simulink model "EE464_HW2"  (R2021b)
settings: Solver=VariableStepAuto  StartTime=0.0  StopTime=0.001  RelTol=1e-3
libraries: spsSeriesRLCBranchLib x7, spsMosfetLib x4, spsVoltageMeasurementLib x4, spsCurrentMeasurementLib x2, spsDiodeLib x2, spsDCVoltageSourceLib x1, spsMultiWindingTransformerLib x1, spspowerguiLib x1
settings Model: Creator=Casper  LastModifiedBy=Casper

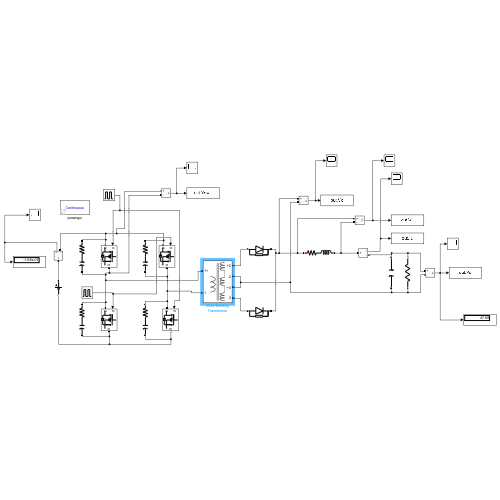
[thumbnail: Simulink's stored preview of the top-level diagram]
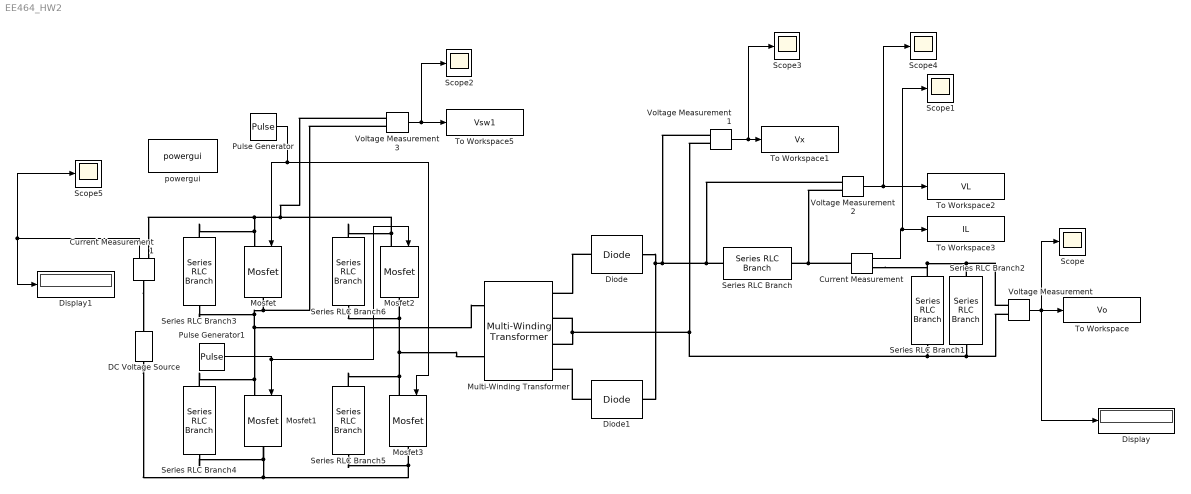
== system EE464_HW2 ==
  Current Measurement : spsCurrentMeasurementLib/Current Measurement  PhasorSimulation=off  OutputType=Complex  PSBequivalent=0
  Current Measurement1 : spsCurrentMeasurementLib/Current Measurement  PhasorSimulation=off  OutputType=Complex  PSBequivalent=0
  DC Voltage Source : spsDCVoltageSourceLib/DC Voltage Source  Amplitude=12  Measurements=None
  Diode : spsDiodeLib/Diode  Ron=0.001  Lon=0  Vf=0.001  IC=0  UseSnubber=0  Rs=500  Cs=250e-9  Measurements=off
  Diode1 : spsDiodeLib/Diode  Ron=0.001  Lon=0  Vf=0.001  IC=0  UseSnubber=0  Rs=500  Cs=250e-9  Measurements=off
  Display : Display
  Display1 : Display
  Mosfet{,1..3} (4 alike) : spsMosfetLib/Mosfet  Ron=0  Lon=0  Rd=0  Vfd=0  IC=0  Rs=inf  Cs=inf  Measurements=off
  Multi-Winding Transformer : spsMultiWindingTransformerLib/Multi-Winding Transformer  LeftWindings=1  RightWindings=2  TappedWindings=no taps  NumberOfTaps=2  SetSaturation=off  Hysteresis=off  DataFile='hysteresis.mat'  Measurements=None  UNITS=SI  NominalPower=[96 100e3]  NominalVoltages="[ 12  60  60 60 ]"  WindingResistances=[0 0 0 0]  WindingInductances=[0 0 0 0]  Rm=Inf  Lm=Inf  Saturation=[0 0;0.3072 8.754e-10;128 1.1088e-09]  BreakLoop=off  DiscreteSolver=Trapezoidal iterative  DataType=on  InitialFlux=0  TransfoNumber=1
      settings: SourceProductBaseCode=PS
  Pulse Generator : DiscretePulseGenerator  PulseType=Time based  Period=1e-5  PulseWidth=40
  Pulse Generator1 : DiscretePulseGenerator  PulseType=Time based  Period=1e-5  PulseWidth=40  PhaseDelay=5e-6
  Scope{,1..5} (6 alike) : Scope
  Series RLC Branch : spsSeriesRLCBranchLib/Series RLC Branch  LConnTagsString=__new0  RConnTagsString=__new0  BranchType=RL  Resistance=1e-10  Inductance=240e-6  SetiL0=off  InitialCurrent=0  Capacitance=1e-6  Setx0=off  InitialVoltage=0  Measurements=None
  Series RLC Branch1 : spsSeriesRLCBranchLib/Series RLC Branch  LConnTagsString=__new0  RConnTagsString=__new0  BranchType=C  Resistance=1  Inductance=1e-3  SetiL0=off  InitialCurrent=0  Capacitance=260.4e-9  Setx0=off  InitialVoltage=0  Measurements=None
  Series RLC Branch2 : spsSeriesRLCBranchLib/Series RLC Branch  LConnTagsString=__new0  RConnTagsString=__new0  BranchType=R  Resistance=24  Inductance=1e-3  SetiL0=off  InitialCurrent=0  Capacitance=1e-6  Setx0=off  InitialVoltage=0  Measurements=None
  Series RLC Branch{3..6} (4 alike) : spsSeriesRLCBranchLib/Series RLC Branch  LConnTagsString=__new0  RConnTagsString=__new0  BranchType=RC  Resistance=0.01  Inductance=1e-3  SetiL0=off  InitialCurrent=0  Capacitance=1e-12  Setx0=off  InitialVoltage=0  Measurements=None
  To Workspace : ToWorkspace  VariableName=Vo  SaveFormat=Timeseries  SampleTime=-1
  To Workspace1 : ToWorkspace  VariableName=Vx  SaveFormat=Timeseries  SampleTime=-1
  To Workspace2 : ToWorkspace  VariableName=VL  SaveFormat=Timeseries  SampleTime=-1
  To Workspace3 : ToWorkspace  VariableName=IL  SaveFormat=Timeseries  SampleTime=-1
  To Workspace5 : ToWorkspace  VariableName=Vsw1  SaveFormat=Timeseries  SampleTime=-1
  Voltage Measurement{,1..3} (4 alike) : spsVoltageMeasurementLib/Voltage Measurement  PhasorSimulation=off  OutputType=Complex  PSBequivalent=0
  powergui : spspowerguiLib/powergui  Priority=1  SimulationMode=Continuous  SampleTime=50e-6  frequency=60  Iterations=50  frequencyindice=0  Pbase=100e6  ErrMax=1e-4  UnitsV=kV  UnitsW=MW  buscounter=0  FunctionMessages=off  echomessages=off  EnableUseOfTLC=off  CurrentSourceSwitches=off  DisableSnubberDevices=off  DisableRonSwitches=off  DisableVfSwitches=off  DisplayEquations=off  AutomaticDiscreteSolvers=off  SolverType=Tustin/Backward Euler (TBE)  Interpol=off  ExternalGateDelay=off  methode=off  Ts=100  x0status=blocks  SPID=on  SwTol=0  HookPort=off  NonlinearTolerance=1e-4  nMaxIteration=100  ContinueOnMaxIteration=off  RestoreLinks=warning  ResistiveCurrentMeasurement=off  Frange=[0:2:500]  Ylog=off  Xlog=on  ShowGrid=off  save=off  variable=ZData  structure=0  ZoomFFT=off  StartTime=0.0  cycles=1  DisplayStyle=1  fundamental=60  FreqAxis=off  MaxFrequency=1000  frequencyindicesteady=1  RmsSteady=1  display=off
  wires:
  Pulse Generator/1 -> Mosfet3/1, Mosfet/1
  Pulse Generator1/1 -> Mosfet2/1, Mosfet1/1
  Voltage Measurement/1 -> Display/1, Scope/1, To Workspace/1
  Current Measurement/1 -> Scope1/1, To Workspace3/1
  Voltage Measurement3/1 -> Scope2/1, To Workspace5/1
  Voltage Measurement1/1 -> Scope3/1, To Workspace1/1
  Voltage Measurement2/1 -> Scope4/1, To Workspace2/1
  Current Measurement1/1 -> Display1/1, Scope5/1
  connections:
  Series RLC Branch6/LConn1 -- Mosfet2/LConn1 -- Voltage Measurement3/LConn1 -- Current Measurement1/RConn1 -- Series RLC Branch3/LConn1 -- Mosfet/LConn1
  Multi-Winding Transformer/LConn1 -- Series RLC Branch4/LConn1 -- Mosfet1/LConn1 -- Series RLC Branch3/RConn1 -- Voltage Measurement3/LConn2 -- Mosfet/RConn1
  Mosfet3/LConn1 -- Series RLC Branch5/LConn1 -- Multi-Winding Transformer/LConn2 -- Series RLC Branch6/RConn1 -- Mosfet2/RConn1
  DC Voltage Source/LConn1 -- Series RLC Branch4/RConn1 -- Mosfet1/RConn1 -- Series RLC Branch5/RConn1 -- Mosfet3/RConn1
  Diode1/LConn1 -- Multi-Winding Transformer/RConn4
  Diode/LConn1 -- Multi-Winding Transformer/RConn1
  Series RLC Branch1/RConn1 -- Voltage Measurement/LConn2 -- Series RLC Branch2/RConn1 -- Voltage Measurement1/LConn2 -- Multi-Winding Transformer/RConn2 -- Multi-Winding Transformer/RConn3
  Diode/RConn1 -- Series RLC Branch/LConn1 -- Voltage Measurement2/LConn1 -- Voltage Measurement1/LConn1 -- Diode1/RConn1
  Series RLC Branch1/LConn1 -- Current Measurement/RConn1 -- Voltage Measurement/LConn1 -- Series RLC Branch2/LConn1
  Voltage Measurement2/LConn2 -- Series RLC Branch/RConn1 -- Current Measurement/LConn1
  Current Measurement1/LConn1 -- DC Voltage Source/RConn1
